simulink model "linear_plant"  (R2019b)
settings: Solver=ode4  StartTime=0.0  StopTime=30.0  FixedStep=1e-4  RelTol=1e-3
settings Model: Creator=Dhruv Laad  LastModifiedBy=Dhruv Laad
settings DebuggingCC: UnderSpecifiedDimensionMsg=warning

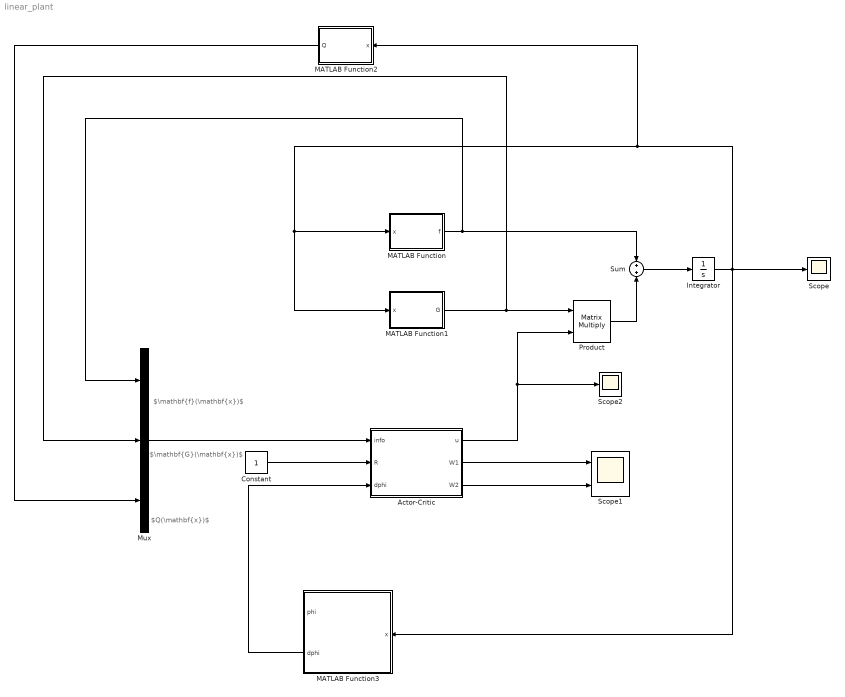
== system linear_plant ==
  note: $Q(\mathbf{x})$
  note: $\mathbf{f}(\mathbf{x})$
  note: $\mathbf{G}(\mathbf{x})$
  Actor-Critic : Subsystem
  Constant : Constant
  Integrator : Integrator  InitialCondition=[10;25;-15]
  MATLAB Function : MATLAB Function  TreatAsAtomicUnit=on
  MATLAB Function1 : MATLAB Function  TreatAsAtomicUnit=on
  MATLAB Function2 : MATLAB Function  TreatAsAtomicUnit=on
  MATLAB Function3 : MATLAB Function  TreatAsAtomicUnit=on
  Mux : Mux  Inputs=3
  Product : Product  Inputs=**  Multiplication=Matrix(*)
  Scope : Scope
  Scope1 : Scope  NumInputPorts=2
  Scope2 : Scope
  Sum : Sum
  wires:
  MATLAB Function/1(f) -> Mux/1, Sum/1
  MATLAB Function1/1(G) -> Mux/2, Product/1
  Product/1 -> Sum/2
  Sum/1 -> Integrator/1
  Actor-Critic/1(u) -> Scope2/1, Product/2
  Integrator/1 -> MATLAB Function3/1(x), Scope/1, MATLAB Function1/1(x), MATLAB Function/1(x), MATLAB Function2/1(x)
  Mux/1 -> Actor-Critic/1(info)
  MATLAB Function2/1(Q) -> Mux/3
  Actor-Critic/2(W1) -> Scope1/1
  Actor-Critic/3(W2) -> Scope1/2
  Constant/1 -> Actor-Critic/2(R)
  MATLAB Function3/2(dphi) -> Actor-Critic/3(dphi)

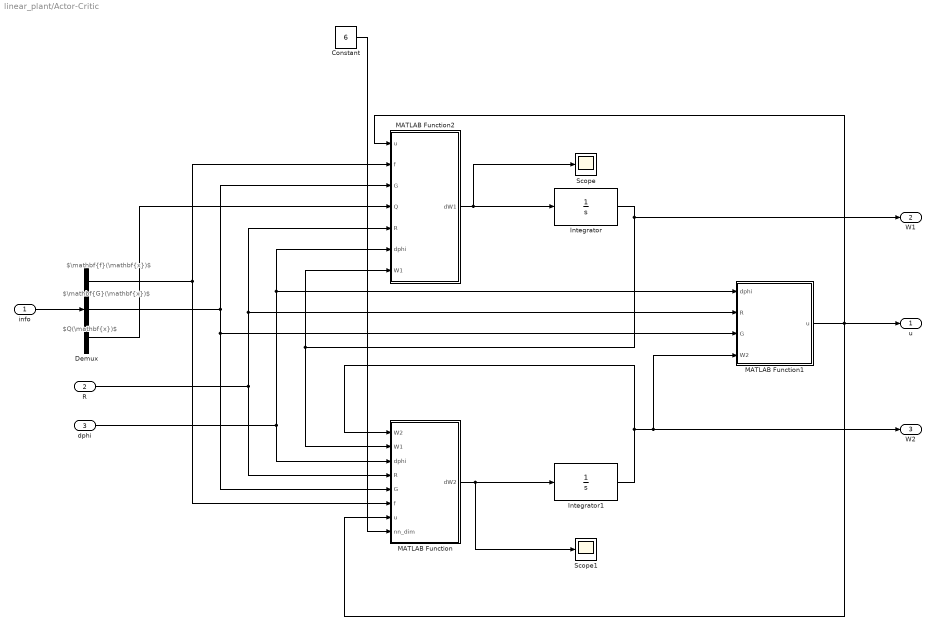
== system linear_plant/Actor-Critic ==
  note: $\mathbf{f}(\mathbf{x})$
  note: $\mathbf{G}(\mathbf{x})$
  note: $Q(\mathbf{x})$
  info : Inport
  R : Inport  Port=2
  dphi : Inport  Port=3
  Constant : Constant  Value=6
  Demux : Demux  Outputs=3
  Integrator : Integrator  InitialCondition=randn(6,1)
  Integrator1 : Integrator  InitialCondition=randn(6,1)
  MATLAB Function : MATLAB Function  TreatAsAtomicUnit=on
  MATLAB Function1 : MATLAB Function  TreatAsAtomicUnit=on
  MATLAB Function2 : MATLAB Function  TreatAsAtomicUnit=on
  Scope : Scope
  Scope1 : Scope
  u : Outport
  W1 : Outport  Port=2
  W2 : Outport  Port=3
  wires:
  info/1 -> Demux/1
  Demux/1 -> MATLAB Function2/2(f), MATLAB Function/6(f)
  Demux/2 -> MATLAB Function1/3(G), MATLAB Function/5(G), MATLAB Function2/3(G)
  Demux/3 -> MATLAB Function2/4(Q)
  R/1 -> MATLAB Function/4(R), MATLAB Function1/2(R), MATLAB Function2/5(R)
  dphi/1 -> MATLAB Function/3(dphi), MATLAB Function2/6(dphi), MATLAB Function1/1(dphi)
  MATLAB Function2/1(dW1) -> Integrator/1, Scope/1
  MATLAB Function/1(dW2) -> Scope1/1, Integrator1/1
  Integrator/1 -> MATLAB Function2/7(W1), MATLAB Function/2(W1), W1/1
  Integrator1/1 -> MATLAB Function/1(W2), MATLAB Function1/4(W2), W2/1
  MATLAB Function1/1(u) -> MATLAB Function/7(u), MATLAB Function2/1(u), u/1
  Constant/1 -> MATLAB Function/8(nn_dim)

== matlab function linear_plant/MATLAB Function1 ==
  data: x input; G output
function G = dyn_G(x)
    G = [0;0;1];

== matlab function linear_plant/MATLAB Function ==
  data: x input; f output
function f = dyn_f(x)
    A = [-1.01887,  0.90506, -0.00215;
          0.82225, -1.07741, -0.17555;
          0      ,  0      , -1];
    f = A*x;

== matlab function linear_plant/Actor-Critic/MATLAB Function2 ==
  data: u input; dW1 output; f input size=3,1; G input size=3,1; Q input; R input; dphi input; W1 input
function dW1 = Critic(u, f, G, Q, R, dphi, W1)
    critic_lr = 0.1;

    sig_2 = dphi*(f + G*u);
    dW1 = -critic_lr*(sig_2/(sig_2'*sig_2 + 1)^2)*(sig_2'*W1 + Q + u'*R*u);

== matlab function linear_plant/Actor-Critic/MATLAB Function ==
  data: W2 input; W1 input; dphi input; R input; G input; f input; u input; dW2 output; nn_dim input
function dW2 = Actor(W2, W1, dphi, R, G, f, u, nn_dim)
    actor_lr = 0.1;
    F2 = 4*eye(nn_dim);
    F1 = 0.1*ones(nn_dim,1);
    
    sig_2 = dphi*(f + G*u);
    D1 = dphi*G*(inv(R))*(G')*dphi';
    m = sig_2/(sig_2'*sig_2 + 1)^2;
    sig2_bar = sig_2/(sig_2'*sig_2 + 1);
    dW2 = -actor_lr*((F2*W2 - F1*sig2_bar'*W1) - 0.25*D1*W2*m'*W1);

== matlab function linear_plant/Actor-Critic/MATLAB Function1 ==
  data: dphi input; R input; u output; G input; W2 input
function u = control_policy(dphi, R, G, W2)
    u = -0.5*(inv(R))*((G)')*(dphi')*W2;

== matlab function linear_plant/MATLAB Function2 ==
  data: x input; Q output
function Q = Q(x)
    Q = x'*x;

== matlab function linear_plant/MATLAB Function3 ==
  data: x input; phi output; dphi output
function [phi, dphi] = basis(x)
    phi = [x(1);x(1)^2;x(2);x(2)^2;x(3);x(3)^2];
    dphi = [1,0,0;2*x(1),0,0;0,1,0;0,2*x(2),0;0,0,1;0,0,2*x(3)];
